simulink model "torqueBalancingStandup"  (Simulink 9.1)
settings: Solver=FixedStepDiscrete  StartTime=0.0  StopTime="Config.SIMULATION_TIME "  FixedStep=Config.Ts  RelTol=1e-3  EnableMultiTasking=on
InitFcn:
  | cd(fileparts(which(bdroot)));
  | initTorqueBalancingStandup;
StopFcn:
  | cd(fileparts(which(bdroot)));
  | stopTorqueBalancingStandup;
undefined symbols (not defined in the file or in its folder): bVectorConstraintsFeet, bVectorConstraintsLegs, Config, ConstraintsMatrixFeet, ConstraintsMatrixLegs, Gain, Reg, ROBOT_DOF, ROBOT_DOF_FOR_SIMULINK, Sat, Sm
libraries: WBToolboxLibrary x95, simulink x4
(part 2 of 2)

== system torqueBalancingStandup/Robot State and References/Select State and References/Visualize Gain Tuning   ==
  smoothingTimeComAndJoints : Inport
  LEFT_RIGHT_FOOT_IN_CONTACT : Inport  Port=2
  impedances : Inport  Port=3
  state : Inport  Port=4
  nu : Inport  Port=5
  Enable : EnablePort
  Demux : Demux  Outputs=2
  Demux1 : Demux  Outputs=Config.numOfJointsForEachControlboard
  Demux2 : Demux  Outputs=Config.numOfJointsForEachControlboard
  Gain : Gain  Gain=180/pi
  Gain1 : Gain  Gain=180/pi
  Impedances(t) : Scope  NumInputPorts=6
  Left right foot in contact : Scope
  Selector1 : Selector  InputPortWidth=6+ROBOT_DOF  IndexOptions=Index vector (dialog)  Indices=[7:6+ROBOT_DOF]  OutputSizes=1
  Selector2 : Selector  InputPortWidth=6+ROBOT_DOF  IndexOptions=Index vector (dialog)  Indices=[1:6]  OutputSizes=1
  jointsSmoothingTime : Scope  NumInputPorts=2
  linear and angular  base velocity : Scope  NumInputPorts=3
  "qjDot(t) " : Scope  NumInputPorts=6
  wires:
  state/1 -> "qjDot(t) "/6, linear and angular  base velocity/3, Impedances(t)/6, jointsSmoothingTime/2  "state"
  LEFT_RIGHT_FOOT_IN_CONTACT/1 -> Left right foot in contact/1  "Left right foot in contact"
  impedances/1 -> Demux1/1
  smoothingTimeComAndJoints/1 -> jointsSmoothingTime/1  "smoothingTimeComAndJoints"
  Demux1/4 -> Impedances(t)/4  "left_leg"
  Demux1/5 -> Impedances(t)/5  "right_leg"
  Demux1/3 -> Impedances(t)/3  "right_arm"
  Demux1/1 -> Impedances(t)/1  "torso"
  Demux1/2 -> Impedances(t)/2  "left_arm"
  Selector1/1 -> Gain/1
  Demux2/4 -> "qjDot(t) "/4  "left_leg"
  Demux2/3 -> "qjDot(t) "/3  "right_arm"
  Demux2/1 -> "qjDot(t) "/1  "torso"
  Demux2/2 -> "qjDot(t) "/2  "left_arm"
  nu/1 -> Selector2/1, Selector1/1
  Selector2/1 -> Demux/1
  Demux/1 -> linear and angular  base velocity/1  "vb"
  Demux/2 -> Gain1/1  "wb"
  Gain/1 -> Demux2/1
  Gain1/1 -> linear and angular  base velocity/2
  Demux2/5 -> "qjDot(t) "/5  "right_leg"

== system torqueBalancingStandup/Robot State and References/State Machine Standup/Compute State Velocity ==
  qj : Inport
  w_H_b : Inport  Port=2
  "feetInContact " : Inport  Port=3
  "state " : Inport  Port=4
  Compute Base Velocity : MATLAB Function  TreatAsAtomicUnit=on
  Fixed Links Jacobians : Subsystem
  Get Measurement : WBToolboxLibrary/wholeBodyStates/Get Measurement  measuredType=Joints Velocity
      settings: SourceProductName=Whole Body Toolbox
  Mux : Mux  Inputs=2
  nu : Outport
  wires:
  Get Measurement/1 -> Mux/2, Compute Base Velocity/4(qjDot)
  Mux/1 -> nu/1
  "feetInContact "/1 -> Compute Base Velocity/3(feetInContact)
  Compute Base Velocity/1(nu_b) -> Mux/1
  Fixed Links Jacobians/1(J_LeftFixed) -> Compute Base Velocity/1(J_LeftFixedLink)
  Fixed Links Jacobians/2(J_RightFixed) -> Compute Base Velocity/2(J_RightFixedLink)
  "state "/1 -> Fixed Links Jacobians/1("state ")
  qj/1 -> Fixed Links Jacobians/2(qj)
  w_H_b/1 -> Fixed Links Jacobians/3(w_H_b)

== system torqueBalancingStandup/Robot State and References/State Machine Standup/Compute base to fixed link transform ==
  qj : Inport
  inertial : Inport  Port=2
  Constant7 : Constant  Value=eye(4)
  "LFoot to base link transform " : Subsystem
  LFoot to world transform (fixed base) : WBToolboxLibrary/wholeBodyModel/Kinematics/Forward Kinematics  frameName=Frames.LEFT_FOOT
      settings: SourceProductName=Whole Body Toolbox
  LLeg to base link transform : Subsystem
  LLeg to world transform (fixed base) : WBToolboxLibrary/wholeBodyModel/Kinematics/Forward Kinematics  frameName=Frames.LEFT_LEG
      settings: SourceProductName=Whole Body Toolbox
  fixed_LFoot_H_b : Outport
  fixed_LLeg_H_b : Outport  Port=2
  wires:
  Constant7/1 -> LLeg to base link transform/4(w_H_base_fixed), "LFoot to base link transform "/4(w_H_base_fixed), LLeg to world transform (fixed base)/1, LFoot to world transform (fixed base)/1
  LLeg to base link transform/1(link_H_b) -> fixed_LLeg_H_b/1
  "LFoot to base link transform "/1(link_H_b) -> fixed_LFoot_H_b/1
  LFoot to world transform (fixed base)/1 -> "LFoot to base link transform "/3(w_H_link)
  LLeg to world transform (fixed base)/1 -> LLeg to base link transform/3(w_H_link)
  qj/1 -> "LFoot to base link transform "/1(qj), LLeg to base link transform/1(qj), LLeg to world transform (fixed base)/2, LFoot to world transform (fixed base)/2
  inertial/1 -> "LFoot to base link transform "/2(inertial), LLeg to base link transform/2(inertial)

== system torqueBalancingStandup/Robot State and References/State Machine Standup/Visualise extrnal wrenches ==
  wL_arm : Inport
  wR_arm : Inport  Port=2
  wL_WBDT : Inport  Port=3
  wR_WBDT : Inport  Port=4
  state : Inport  Port=5
  Enable : EnablePort
  Compute current threshold : MATLAB Function  TreatAsAtomicUnit=on
  Sum : Sum  Inputs=++|
  Sum1 : Sum  Inputs=++|
  left arm ext wrench : Scope  NumInputPorts=3
  left foot ext wrench : Scope  NumInputPorts=3
  right arm ext wrench : Scope  NumInputPorts=3
  right foot ext wrench : Scope  NumInputPorts=3
  sum feet ext wrench : Scope  NumInputPorts=3
  wires:
  wR_WBDT/1 -> Sum/2, right foot ext wrench/1  "wR_WBDT"
  wL_WBDT/1 -> Sum/1, left foot ext wrench/1  "wL_WBDT"
  wR_arm/1 -> right arm ext wrench/1
  wL_arm/1 -> left arm ext wrench/1
  state/1 -> Compute current threshold/1(state), sum feet ext wrench/3, right foot ext wrench/3, left foot ext wrench/3, right arm ext wrench/3, left arm ext wrench/3
  Sum/1 -> sum feet ext wrench/1
  Sum1/1 -> sum feet ext wrench/2
  Compute current threshold/3(thresholdContactLeftFoot) -> left foot ext wrench/2, Sum1/1
  Compute current threshold/4(thresholdContactRightFoot) -> right foot ext wrench/2, Sum1/2
  Compute current threshold/1(thresholdContactLeftHand) -> left arm ext wrench/2
  Compute current threshold/2(thresholdContactRightHand) -> right arm ext wrench/2

== system torqueBalancingStandup/Robot State and References/State Machine Standup/xCom ==
  w_H_b : Inport
  qj : Inport  Port=2
  CoM : WBToolboxLibrary/wholeBodyModel/Kinematics/Forward Kinematics  frameName=Frames.COM
      settings: SourceProductName=Whole Body Toolbox
  "CoM6D ->  CoMXYZ2" : Selector  NumberOfDimensions=2  InputPortWidth=7  IndexOptions=Index vector (dialog),Index vector (dialog)  Indices=[1 2 3],[4]  OutputSizes=1,1
  xCoM : Outport
  wires:
  qj/1 -> CoM/2
  "CoM6D ->  CoMXYZ2"/1 -> xCoM/1
  CoM/1 -> "CoM6D ->  CoMXYZ2"/1
  w_H_b/1 -> CoM/1

== system torqueBalancingStandup/controller_QP/Compute angular momentum integral/Compute base to fixed link transform ==
  qj : Inport
  inertial : Inport  Port=2
  Constant7 : Constant  Value=eye(4)
  "LFoot to base link transform " : Subsystem
  LFoot to world transform (fixed base) : WBToolboxLibrary/wholeBodyModel/Kinematics/Forward Kinematics  frameName=Frames.LEFT_FOOT
      settings: SourceProductName=Whole Body Toolbox
  LLeg to base link transform : Subsystem
  LLeg to world transform (fixed base) : WBToolboxLibrary/wholeBodyModel/Kinematics/Forward Kinematics  frameName=Frames.LEFT_LEG
      settings: SourceProductName=Whole Body Toolbox
  fixed_LLeg_H_b : Outport
  fixed_LFoot_H_b : Outport  Port=2
  wires:
  Constant7/1 -> LLeg to base link transform/4(w_H_base_fixed), "LFoot to base link transform "/4(w_H_base_fixed), LLeg to world transform (fixed base)/1, LFoot to world transform (fixed base)/1
  LLeg to base link transform/1(link_H_b) -> fixed_LLeg_H_b/1
  "LFoot to base link transform "/1(link_H_b) -> fixed_LFoot_H_b/1
  LFoot to world transform (fixed base)/1 -> "LFoot to base link transform "/3(w_H_link)
  LLeg to world transform (fixed base)/1 -> LLeg to base link transform/3(w_H_link)
  qj/1 -> "LFoot to base link transform "/1(qj), LLeg to base link transform/1(qj), LLeg to world transform (fixed base)/2, LFoot to world transform (fixed base)/2
  inertial/1 -> "LFoot to base link transform "/2(inertial), LLeg to base link transform/2(inertial)

== system torqueBalancingStandup/controller_QP/Compute angular momentum integral/Fixed Links Jacobians ==
  "legsInContact " : Inport
  qj : Inport  Port=2
  w_H_b : Inport  Port=3
  " " : WBToolboxLibrary/wholeBodyModel/Jacobians/Jacobian  frameName=Frames.LEFT_LEG
      settings: SourceProductName=Whole Body Toolbox
  "  " : WBToolboxLibrary/wholeBodyModel/Jacobians/Jacobian  frameName=Frames.RIGHT_LEG
      settings: SourceProductName=Whole Body Toolbox
  "   " : WBToolboxLibrary/wholeBodyModel/Jacobians/Jacobian  frameName=Frames.RIGHT_FOOT
      settings: SourceProductName=Whole Body Toolbox
  "       " : WBToolboxLibrary/wholeBodyModel/Jacobians/Jacobian  frameName=Frames.LEFT_FOOT
      settings: SourceProductName=Whole Body Toolbox
  Switch1 : Switch  Criteria=u2 > Threshold  Threshold=0.1
  Switch2 : Switch  Criteria=u2 > Threshold  Threshold=0.1
  J_LeftFixed : Outport
  J_RIghtFixed : Outport  Port=2
  wires:
  Switch2/1 -> J_RIghtFixed/1
  " "/1 -> Switch1/1
  "       "/1 -> Switch1/3
  "   "/1 -> Switch2/3
  "  "/1 -> Switch2/1
  Switch1/1 -> J_LeftFixed/1
  qj/1 -> "   "/2, "  "/2, "       "/2, " "/2
  w_H_b/1 -> "   "/1, " "/1, "       "/1, "  "/1
  "legsInContact "/1 -> Switch2/2, Switch1/2

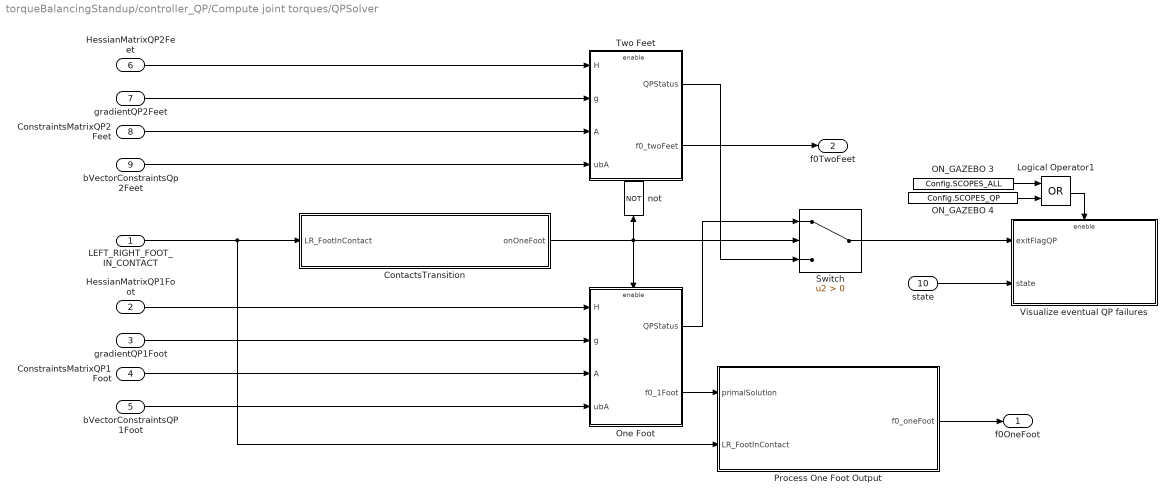
== system torqueBalancingStandup/controller_QP/Compute joint torques/QPSolver ==
  LEFT_RIGHT_FOOT_IN_CONTACT : Inport
  HessianMatrixQP1Foot : Inport  Port=2
  gradientQP1Foot : Inport  Port=3
  ConstraintsMatrixQP1Foot : Inport  Port=4
  bVectorConstraintsQP1Foot : Inport  Port=5
  HessianMatrixQP2Feet : Inport  Port=6
  gradientQP2Feet : Inport  Port=7
  ConstraintsMatrixQP2Feet : Inport  Port=8
  bVectorConstraintsQp2Feet : Inport  Port=9
  state : Inport  Port=10
  ContactsTransition : MATLAB Function  TreatAsAtomicUnit=on
  Logical Operator1 : Logic  Operator=OR  AllPortsSameDT=off  OutDataTypeStr=boolean
  ON_GAZEBO 3 : Constant  Value=Config.SCOPES_ALL
  ON_GAZEBO 4 : Constant  Value=Config.SCOPES_QP
  One Foot : Subsystem  TreatAsAtomicUnit=on
  Process One Foot Output : MATLAB Function  TreatAsAtomicUnit=on
  Switch : Switch  Criteria=u2 > Threshold
  Two Feet : Subsystem  TreatAsAtomicUnit=on
  Visualize eventual QP failures : Subsystem
  not : Logic  Operator=NOT  IconShape=distinctive  AllPortsSameDT=off  OutDataTypeStr=boolean
  f0OneFoot : Outport
  f0TwoFeet : Outport  Port=2
  wires:
  Logical Operator1/1 -> Visualize eventual QP failures/Enable
  state/1 -> Visualize eventual QP failures/2(state)
  LEFT_RIGHT_FOOT_IN_CONTACT/1 -> Process One Foot Output/2(LR_FootInContact), ContactsTransition/1(LR_FootInContact)
  ON_GAZEBO 3/1 -> Logical Operator1/1
  ON_GAZEBO 4/1 -> Logical Operator1/2
  HessianMatrixQP1Foot/1 -> One Foot/1(H)
  bVectorConstraintsQp2Feet/1 -> Two Feet/4(ubA)
  gradientQP1Foot/1 -> One Foot/2(g)
  ConstraintsMatrixQP1Foot/1 -> One Foot/3(A)
  gradientQP2Feet/1 -> Two Feet/2(g)
  ConstraintsMatrixQP2Feet/1 -> Two Feet/3(A)
  not/1 -> Two Feet/Enable
  ContactsTransition/1(onOneFoot) -> One Foot/Enable, Switch/2, not/1
  bVectorConstraintsQP1Foot/1 -> One Foot/4(ubA)
  HessianMatrixQP2Feet/1 -> Two Feet/1(H)
  One Foot/2(f0_1Foot) -> Process One Foot Output/1(primalSolution)
  Process One Foot Output/1(f0_oneFoot) -> f0OneFoot/1
  One Foot/1(QPStatus) -> Switch/1
  Two Feet/1(QPStatus) -> Switch/3
  Switch/1 -> Visualize eventual QP failures/1(exitFlagQP)
  Two Feet/2(f0_twoFeet) -> f0TwoFeet/1

== system torqueBalancingStandup/controller_QP/Compute joint torques (motor reflected inertia)/Check the contribution of feedforward ==
  feedForward : Inport
  u : Inport  Port=2
  Enable : EnablePort
  Demux1 : Demux  Outputs=Config.numOfJointsForEachControlboard
  Demux10 : Demux  Outputs=Config.numOfJointsForEachControlboard
  Demux2 : Demux  Outputs=Config.numOfJointsForEachControlboard
  Sum : Sum  Inputs=|+-
  feedforward_only : Scope  NumInputPorts=5
  u_only : Scope  NumInputPorts=5
  u_with_feedforward : Scope  NumInputPorts=5
  wires:
  Demux10/5 -> u_with_feedforward/5  "right_leg"
  Demux10/2 -> u_with_feedforward/2  "left_arm"
  Demux10/3 -> u_with_feedforward/3  "right_arm"
  Demux10/1 -> u_with_feedforward/1  "torso"
  Demux10/4 -> u_with_feedforward/4  "left_leg"
  Sum/1 -> Demux10/1  "u_with_feedForward"
  feedForward/1 -> Demux1/1, Sum/2
  Demux1/4 -> feedforward_only/4  "left_leg"
  Demux1/5 -> feedforward_only/5  "right_leg"
  Demux1/2 -> feedforward_only/2  "left_arm"
  Demux1/1 -> feedforward_only/1  "torso"
  Demux1/3 -> feedforward_only/3  "right_arm"
  Demux2/4 -> u_only/4  "left_leg"
  Demux2/3 -> u_only/3  "right_arm"
  Demux2/5 -> u_only/5  "right_leg"
  Demux2/2 -> u_only/2  "left_arm"
  u/1 -> Demux2/1, Sum/1
  Demux2/1 -> u_only/1  "torso"

== system torqueBalancingStandup/Robot State and References/Internal Coordinator/Base to fixed_link/LFoot to base link transform  ==
  qj : Inport
  inertial : Inport  Port=2
  w_H_link : Inport  Port=3
  w_H_base_fixed : Inport  Port=4
  Fixed base to imu transform : WBToolboxLibrary/wholeBodyModel/Kinematics/Forward Kinematics  frameName=Frames.IMU
      settings: SourceProductName=Whole Body Toolbox
  Fixed base to root link transform : WBToolboxLibrary/wholeBodyModel/Kinematics/Forward Kinematics  frameName=Frames.BASE
      settings: SourceProductName=Whole Body Toolbox
  Inv\* : Product  Inputs=/*  Multiplication=Matrix(*)
  "Inv\\*  " : Product  Inputs=/*  Multiplication=Matrix(*)
  Neck Position : WBToolboxLibrary/Utilities/Yarp Read  portName=Ports.NECK_POS  signalSize=6  timeout=0.5  blocking=off  timestamp=off  autoconnect=on  errorOnConnection=off
      settings: SourceProductName=Whole Body Toolbox
  Switch6 : Switch  Criteria=u2 > Threshold
  USE_IMU4EST_BASE : Constant  Value=Config.USE_IMU4EST_BASE
  fromImuToHomogeousTransformFCN : MATLAB Function  TreatAsAtomicUnit=on
  holder 1 : WBToolboxLibrary/Utilities/holder 
      settings: SourceProductName=Whole Body Toolbox
  holder 2 : WBToolboxLibrary/Utilities/holder 
      settings: SourceProductName=Whole Body Toolbox
  neck transform : Subsystem
  link_H_b : Outport
  wires:
  Switch6/1 -> link_H_b/1
  "Inv\\*  "/1 -> Switch6/3, fromImuToHomogeousTransformFCN/3(link_H_base)  "link_H_root"
  USE_IMU4EST_BASE/1 -> Switch6/2
  Inv\*/1 -> fromImuToHomogeousTransformFCN/1(imu_H_link), holder 1/1  "imu_H_link"
  holder 2/1 -> fromImuToHomogeousTransformFCN/4(inertial_0)
  Fixed base to imu transform/1 -> Inv\*/1
  holder 1/1 -> fromImuToHomogeousTransformFCN/2(imu_H_link_0)
  qj/1 -> Fixed base to imu transform/2, Fixed base to root link transform/2
  fromImuToHomogeousTransformFCN/1(w_H_b) -> Switch6/1
  Fixed base to root link transform/1 -> "Inv\\*  "/2
  inertial/1 -> holder 2/1, fromImuToHomogeousTransformFCN/5(inertial)
  Neck Position/1 -> neck transform/1(neck port)
  neck transform/1(neck position) -> fromImuToHomogeousTransformFCN/6(neck_pos)
  w_H_link/1 -> "Inv\\*  "/1, Inv\*/2
  w_H_base_fixed/1 -> Fixed base to root link transform/1, Fixed base to imu transform/1

== system torqueBalancingStandup/Robot State and References/Internal Coordinator/Compute State Velocity/Feet Jacobians ==
  qj : Inport
  w_H_b : Inport  Port=2
  Jacobian LFoot : WBToolboxLibrary/wholeBodyModel/Jacobians/Jacobian  frameName=Frames.LEFT_FOOT
      settings: SourceProductName=Whole Body Toolbox
  Jacobian RFoot : WBToolboxLibrary/wholeBodyModel/Jacobians/Jacobian  frameName=Frames.RIGHT_FOOT
      settings: SourceProductName=Whole Body Toolbox
  J_LFoot : Outport
  J_RFoot : Outport  Port=2
  wires:
  Jacobian LFoot/1 -> J_LFoot/1
  Jacobian RFoot/1 -> J_RFoot/1
  w_H_b/1 -> Jacobian RFoot/1, Jacobian LFoot/1
  qj/1 -> Jacobian LFoot/2, Jacobian RFoot/2

== system torqueBalancingStandup/Robot State and References/State Machine Standup/Compute State Velocity/Fixed Links Jacobians ==
  "state " : Inport
  qj : Inport  Port=2
  w_H_b : Inport  Port=3
  " " : WBToolboxLibrary/wholeBodyModel/Jacobians/Jacobian  frameName=Frames.LEFT_LEG
      settings: SourceProductName=Whole Body Toolbox
  "  " : WBToolboxLibrary/wholeBodyModel/Jacobians/Jacobian  frameName=Frames.RIGHT_LEG
      settings: SourceProductName=Whole Body Toolbox
  "   " : WBToolboxLibrary/wholeBodyModel/Jacobians/Jacobian  frameName=Frames.RIGHT_FOOT
      settings: SourceProductName=Whole Body Toolbox
  "       " : WBToolboxLibrary/wholeBodyModel/Jacobians/Jacobian  frameName=Frames.LEFT_FOOT
      settings: SourceProductName=Whole Body Toolbox
  Constant : Constant  Value=Config.iCubStandUp
  Legs in Contact : MATLAB Function  TreatAsAtomicUnit=on
  Switch1 : Switch  Criteria=u2 > Threshold  Threshold=0.1
  Switch2 : Switch  Criteria=u2 > Threshold  Threshold=0.1
  J_LeftFixed : Outport
  J_RightFixed : Outport  Port=2
  wires:
  Switch2/1 -> J_RightFixed/1
  Legs in Contact/1(legsInContact) -> Switch2/2, Switch1/2
  " "/1 -> Switch1/1
  "       "/1 -> Switch1/3
  "   "/1 -> Switch2/3
  "  "/1 -> Switch2/1
  "state "/1 -> Legs in Contact/2(state)
  Constant/1 -> Legs in Contact/1(icubStandup)
  Switch1/1 -> J_LeftFixed/1
  qj/1 -> "   "/2, "  "/2, "       "/2, " "/2
  w_H_b/1 -> "   "/1, " "/1, "       "/1, "  "/1

== system torqueBalancingStandup/Robot State and References/State Machine Standup/Compute base to fixed link transform/LFoot to base link transform  ==
  qj : Inport
  inertial : Inport  Port=2
  w_H_link : Inport  Port=3
  w_H_base_fixed : Inport  Port=4
  Fixed base to imu transform : WBToolboxLibrary/wholeBodyModel/Kinematics/Forward Kinematics  frameName=Frames.IMU
      settings: SourceProductName=Whole Body Toolbox
  Fixed base to root link transform : WBToolboxLibrary/wholeBodyModel/Kinematics/Forward Kinematics  frameName=Frames.BASE
      settings: SourceProductName=Whole Body Toolbox
  Inv\* : Product  Inputs=/*  Multiplication=Matrix(*)
  "Inv\\*  " : Product  Inputs=/*  Multiplication=Matrix(*)
  Neck Position : WBToolboxLibrary/Utilities/Yarp Read  portName=Ports.NECK_POS  signalSize=6  timeout=0.5  blocking=off  timestamp=off  autoconnect=on  errorOnConnection=off
      settings: SourceProductName=Whole Body Toolbox
  Switch6 : Switch  Criteria=u2 > Threshold
  USE_IMU4EST_BASE : Constant  Value=Config.USE_IMU4EST_BASE
  fromImuToHomogeousTransformFCN : MATLAB Function  TreatAsAtomicUnit=on
  holder 1 : WBToolboxLibrary/Utilities/holder 
      settings: SourceProductName=Whole Body Toolbox
  holder 2 : WBToolboxLibrary/Utilities/holder 
      settings: SourceProductName=Whole Body Toolbox
  neck transform : Subsystem
  link_H_b : Outport
  wires:
  Switch6/1 -> link_H_b/1
  "Inv\\*  "/1 -> Switch6/3, fromImuToHomogeousTransformFCN/3(link_H_base)  "link_H_root"
  USE_IMU4EST_BASE/1 -> Switch6/2
  Inv\*/1 -> fromImuToHomogeousTransformFCN/1(imu_H_link), holder 1/1  "imu_H_link"
  holder 2/1 -> fromImuToHomogeousTransformFCN/4(inertial_0)
  Fixed base to imu transform/1 -> Inv\*/1
  holder 1/1 -> fromImuToHomogeousTransformFCN/2(imu_H_link_0)
  qj/1 -> Fixed base to imu transform/2, Fixed base to root link transform/2
  fromImuToHomogeousTransformFCN/1(w_H_b) -> Switch6/1
  Fixed base to root link transform/1 -> "Inv\\*  "/2
  inertial/1 -> holder 2/1, fromImuToHomogeousTransformFCN/5(inertial)
  Neck Position/1 -> neck transform/1(neck port)
  neck transform/1(neck position) -> fromImuToHomogeousTransformFCN/6(neck_pos)
  w_H_link/1 -> "Inv\\*  "/1, Inv\*/2
  w_H_base_fixed/1 -> Fixed base to root link transform/1, Fixed base to imu transform/1

== system torqueBalancingStandup/Robot State and References/State Machine Standup/Compute base to fixed link transform/LLeg to base link transform ==
  qj : Inport
  inertial : Inport  Port=2
  w_H_link : Inport  Port=3
  w_H_base_fixed : Inport  Port=4
  Fixed base to imu transform : WBToolboxLibrary/wholeBodyModel/Kinematics/Forward Kinematics  frameName=Frames.IMU
      settings: SourceProductName=Whole Body Toolbox
  Fixed base to root link transform : WBToolboxLibrary/wholeBodyModel/Kinematics/Forward Kinematics  frameName=Frames.BASE
      settings: SourceProductName=Whole Body Toolbox
  Inv\* : Product  Inputs=/*  Multiplication=Matrix(*)
  "Inv\\*  " : Product  Inputs=/*  Multiplication=Matrix(*)
  Neck Position : WBToolboxLibrary/Utilities/Yarp Read  portName=Ports.NECK_POS  signalSize=6  timeout=0.5  blocking=off  timestamp=off  autoconnect=on  errorOnConnection=off
      settings: SourceProductName=Whole Body Toolbox
  Switch6 : Switch  Criteria=u2 > Threshold
  USE_IMU4EST_BASE : Constant  Value=Config.USE_IMU4EST_BASE
  fromImuToHomogeousTransformFCN : MATLAB Function  TreatAsAtomicUnit=on
  holder 1 : WBToolboxLibrary/Utilities/holder 
      settings: SourceProductName=Whole Body Toolbox
  holder 2 : WBToolboxLibrary/Utilities/holder 
      settings: SourceProductName=Whole Body Toolbox
  neck transform : Subsystem
  link_H_b : Outport
  wires:
  Switch6/1 -> link_H_b/1
  "Inv\\*  "/1 -> Switch6/3, fromImuToHomogeousTransformFCN/3(link_H_base)  "link_H_root"
  USE_IMU4EST_BASE/1 -> Switch6/2
  Inv\*/1 -> fromImuToHomogeousTransformFCN/1(imu_H_link), holder 1/1  "imu_H_link"
  holder 2/1 -> fromImuToHomogeousTransformFCN/4(inertial_0)
  Fixed base to imu transform/1 -> Inv\*/1
  holder 1/1 -> fromImuToHomogeousTransformFCN/2(imu_H_link_0)
  qj/1 -> Fixed base to imu transform/2, Fixed base to root link transform/2
  fromImuToHomogeousTransformFCN/1(w_H_b) -> Switch6/1
  Fixed base to root link transform/1 -> "Inv\\*  "/2
  inertial/1 -> holder 2/1, fromImuToHomogeousTransformFCN/5(inertial)
  Neck Position/1 -> neck transform/1(neck port)
  neck transform/1(neck position) -> fromImuToHomogeousTransformFCN/6(neck_pos)
  w_H_link/1 -> "Inv\\*  "/1, Inv\*/2
  w_H_base_fixed/1 -> Fixed base to root link transform/1, Fixed base to imu transform/1

== system torqueBalancingStandup/controller_QP/Compute angular momentum integral/Compute base to fixed link transform/LFoot to base link transform  ==
  qj : Inport
  inertial : Inport  Port=2
  w_H_link : Inport  Port=3
  w_H_base_fixed : Inport  Port=4
  Fixed base to imu transform : WBToolboxLibrary/wholeBodyModel/Kinematics/Forward Kinematics  frameName=Frames.IMU
      settings: SourceProductName=Whole Body Toolbox
  Fixed base to root link transform : WBToolboxLibrary/wholeBodyModel/Kinematics/Forward Kinematics  frameName=Frames.BASE
      settings: SourceProductName=Whole Body Toolbox
  Inv\* : Product  Inputs=/*  Multiplication=Matrix(*)
  "Inv\\*  " : Product  Inputs=/*  Multiplication=Matrix(*)
  Neck Position : WBToolboxLibrary/Utilities/Yarp Read  portName=Ports.NECK_POS  signalSize=6  timeout=0.5  blocking=off  timestamp=off  autoconnect=on  errorOnConnection=off
      settings: SourceProductName=Whole Body Toolbox
  Switch6 : Switch  Criteria=u2 > Threshold
  USE_IMU4EST_BASE : Constant  Value=Config.USE_IMU4EST_BASE
  fromImuToHomogeousTransformFCN : MATLAB Function  TreatAsAtomicUnit=on
  holder 1 : WBToolboxLibrary/Utilities/holder 
      settings: SourceProductName=Whole Body Toolbox
  holder 2 : WBToolboxLibrary/Utilities/holder 
      settings: SourceProductName=Whole Body Toolbox
  neck transform : Subsystem
  link_H_b : Outport
  wires:
  Switch6/1 -> link_H_b/1
  "Inv\\*  "/1 -> Switch6/3, fromImuToHomogeousTransformFCN/3(link_H_base)  "link_H_root"
  USE_IMU4EST_BASE/1 -> Switch6/2
  Inv\*/1 -> fromImuToHomogeousTransformFCN/1(imu_H_link), holder 1/1  "imu_H_link"
  holder 2/1 -> fromImuToHomogeousTransformFCN/4(inertial_0)
  Fixed base to imu transform/1 -> Inv\*/1
  holder 1/1 -> fromImuToHomogeousTransformFCN/2(imu_H_link_0)
  qj/1 -> Fixed base to imu transform/2, Fixed base to root link transform/2
  fromImuToHomogeousTransformFCN/1(w_H_b) -> Switch6/1
  Fixed base to root link transform/1 -> "Inv\\*  "/2
  inertial/1 -> holder 2/1, fromImuToHomogeousTransformFCN/5(inertial)
  Neck Position/1 -> neck transform/1(neck port)
  neck transform/1(neck position) -> fromImuToHomogeousTransformFCN/6(neck_pos)
  w_H_link/1 -> "Inv\\*  "/1, Inv\*/2
  w_H_base_fixed/1 -> Fixed base to root link transform/1, Fixed base to imu transform/1

== system torqueBalancingStandup/controller_QP/Compute angular momentum integral/Compute base to fixed link transform/LLeg to base link transform ==
  qj : Inport
  inertial : Inport  Port=2
  w_H_link : Inport  Port=3
  w_H_base_fixed : Inport  Port=4
  Fixed base to imu transform : WBToolboxLibrary/wholeBodyModel/Kinematics/Forward Kinematics  frameName=Frames.IMU
      settings: SourceProductName=Whole Body Toolbox
  Fixed base to root link transform : WBToolboxLibrary/wholeBodyModel/Kinematics/Forward Kinematics  frameName=Frames.BASE
      settings: SourceProductName=Whole Body Toolbox
  Inv\* : Product  Inputs=/*  Multiplication=Matrix(*)
  "Inv\\*  " : Product  Inputs=/*  Multiplication=Matrix(*)
  Neck Position : WBToolboxLibrary/Utilities/Yarp Read  portName=Ports.NECK_POS  signalSize=6  timeout=0.5  blocking=off  timestamp=off  autoconnect=on  errorOnConnection=off
      settings: SourceProductName=Whole Body Toolbox
  Switch6 : Switch  Criteria=u2 > Threshold
  USE_IMU4EST_BASE : Constant  Value=Config.USE_IMU4EST_BASE
  fromImuToHomogeousTransformFCN : MATLAB Function  TreatAsAtomicUnit=on
  holder 1 : WBToolboxLibrary/Utilities/holder 
      settings: SourceProductName=Whole Body Toolbox
  holder 2 : WBToolboxLibrary/Utilities/holder 
      settings: SourceProductName=Whole Body Toolbox
  neck transform : Subsystem
  link_H_b : Outport
  wires:
  Switch6/1 -> link_H_b/1
  "Inv\\*  "/1 -> Switch6/3, fromImuToHomogeousTransformFCN/3(link_H_base)  "link_H_root"
  USE_IMU4EST_BASE/1 -> Switch6/2
  Inv\*/1 -> fromImuToHomogeousTransformFCN/1(imu_H_link), holder 1/1  "imu_H_link"
  holder 2/1 -> fromImuToHomogeousTransformFCN/4(inertial_0)
  Fixed base to imu transform/1 -> Inv\*/1
  holder 1/1 -> fromImuToHomogeousTransformFCN/2(imu_H_link_0)
  qj/1 -> Fixed base to imu transform/2, Fixed base to root link transform/2
  fromImuToHomogeousTransformFCN/1(w_H_b) -> Switch6/1
  Fixed base to root link transform/1 -> "Inv\\*  "/2
  inertial/1 -> holder 2/1, fromImuToHomogeousTransformFCN/5(inertial)
  Neck Position/1 -> neck transform/1(neck port)
  neck transform/1(neck position) -> fromImuToHomogeousTransformFCN/6(neck_pos)
  w_H_link/1 -> "Inv\\*  "/1, Inv\*/2
  w_H_base_fixed/1 -> Fixed base to root link transform/1, Fixed base to imu transform/1

== system torqueBalancingStandup/controller_QP/Compute joint torques/QPSolver/One Foot ==
  H : Inport
  g : Inport  Port=2
  A : Inport  Port=3
  ubA : Inport  Port=4
  Enable : EnablePort
  Analytical Solution One Foot (unconstrained) : MATLAB Function  TreatAsAtomicUnit=on
  Match Signal Sizes1 : WBToolboxLibrary/Utilities/Match Signal Sizes
      settings: SourceProductName=Whole Body Toolbox
  Process QP output : MATLAB Function  TreatAsAtomicUnit=on
  QP Two Feet : WBToolboxLibrary/Utilities/QP  lbA=off  ubA=on  lb=off  ub=off  computeObjVal=off  stopIfFails=off
      settings: SourceProductName=Whole Body Toolbox
  QPStatus : Outport
  f0_1Foot : Outport  Port=2
  wires:
  H/1 -> Analytical Solution One Foot (unconstrained)/1(H), QP Two Feet/1
  ubA/1 -> QP Two Feet/4
  A/1 -> QP Two Feet/3
  QP Two Feet/2 -> Process QP output/3(QPStatus), QPStatus/1
  QP Two Feet/1 -> Match Signal Sizes1/2
  g/1 -> Analytical Solution One Foot (unconstrained)/2(g), Match Signal Sizes1/1, QP Two Feet/2
  Match Signal Sizes1/1 -> Process QP output/2(primalSolution)
  Analytical Solution One Foot (unconstrained)/1(analyticalSolution) -> Process QP output/1(analyticalSolution)
  Process QP output/1(f0) -> f0_1Foot/1

== system torqueBalancingStandup/controller_QP/Compute joint torques/QPSolver/Two Feet ==
  H : Inport
  g : Inport  Port=2
  A : Inport  Port=3
  ubA : Inport  Port=4
  Enable : EnablePort
  Analytical Solution Two Feet (unconstrained) : MATLAB Function  TreatAsAtomicUnit=on
  Match Signal Sizes : WBToolboxLibrary/Utilities/Match Signal Sizes
      settings: SourceProductName=Whole Body Toolbox
  Process QP output : MATLAB Function  TreatAsAtomicUnit=on
  QP Two Feet : WBToolboxLibrary/Utilities/QP  lbA=off  ubA=on  lb=off  ub=off  computeObjVal=off  stopIfFails=off
      settings: SourceProductName=Whole Body Toolbox
  QPStatus : Outport
  f0_twoFeet : Outport  Port=2
  wires:
  H/1 -> QP Two Feet/1, Analytical Solution Two Feet (unconstrained)/1(H)
  ubA/1 -> QP Two Feet/4
  A/1 -> QP Two Feet/3
  g/1 -> Analytical Solution Two Feet (unconstrained)/2(g), Match Signal Sizes/1, QP Two Feet/2
  QP Two Feet/2 -> QPStatus/1, Process QP output/3(QPStatus)
  QP Two Feet/1 -> Match Signal Sizes/2
  Match Signal Sizes/1 -> Process QP output/2(primalSolution)
  Analytical Solution Two Feet (unconstrained)/1(analyticalSolution) -> Process QP output/1(analyticalSolution)
  Process QP output/1(f0) -> f0_twoFeet/1

== system torqueBalancingStandup/controller_QP/Compute joint torques/QPSolver/Visualize eventual QP failures ==
  exitFlagQP : Inport
  state : Inport  Port=2
  Enable : EnablePort
  "QP status (0: no failure, 1: not using)" : Scope  NumInputPorts=2
  wires:
  exitFlagQP/1 -> "QP status (0: no failure, 1: not using)"/1  "exitFlagQP"
  state/1 -> "QP status (0: no failure, 1: not using)"/2

== system torqueBalancingStandup/Robot State and References/Internal Coordinator/Base to fixed_link/LFoot to base link transform /neck transform ==
  neck port : Inport
  Constant : Constant  Value=zeros(3,1)
  Gain : Gain  Gain=pi/180
  Selector1 : Selector  InputPortWidth=6  IndexOptions=Index vector (dialog)  Indices=[1:3]  OutputSizes=1
  Switch : Switch  Criteria=u2 > Threshold
  USE_IMU4EST_BASE1 : Constant  Value=Config.CORRECT_NECK_IMU
  neck position : Outport
  wires:
  neck port/1 -> Gain/1
  USE_IMU4EST_BASE1/1 -> Switch/2
  Switch/1 -> neck position/1
  Gain/1 -> Selector1/1
  Constant/1 -> Switch/3
  Selector1/1 -> Switch/1  "neck pos"

== system torqueBalancingStandup/Robot State and References/State Machine Standup/Compute base to fixed link transform/LFoot to base link transform /neck transform ==
  neck port : Inport
  Constant : Constant  Value=zeros(3,1)
  Gain : Gain  Gain=pi/180
  Selector1 : Selector  InputPortWidth=6  IndexOptions=Index vector (dialog)  Indices=[1:3]  OutputSizes=1
  Switch : Switch  Criteria=u2 > Threshold
  USE_IMU4EST_BASE1 : Constant  Value=Config.CORRECT_NECK_IMU
  neck position : Outport
  wires:
  neck port/1 -> Gain/1
  USE_IMU4EST_BASE1/1 -> Switch/2
  Switch/1 -> neck position/1
  Gain/1 -> Selector1/1
  Constant/1 -> Switch/3
  Selector1/1 -> Switch/1  "neck pos"

== system torqueBalancingStandup/Robot State and References/State Machine Standup/Compute base to fixed link transform/LLeg to base link transform/neck transform ==
  neck port : Inport
  Constant : Constant  Value=zeros(3,1)
  Gain : Gain  Gain=pi/180
  Selector1 : Selector  InputPortWidth=6  IndexOptions=Index vector (dialog)  Indices=[1:3]  OutputSizes=1
  Switch : Switch  Criteria=u2 > Threshold
  USE_IMU4EST_BASE1 : Constant  Value=Config.CORRECT_NECK_IMU
  neck position : Outport
  wires:
  neck port/1 -> Gain/1
  USE_IMU4EST_BASE1/1 -> Switch/2
  Switch/1 -> neck position/1
  Gain/1 -> Selector1/1
  Constant/1 -> Switch/3
  Selector1/1 -> Switch/1  "neck pos"

== system torqueBalancingStandup/controller_QP/Compute angular momentum integral/Compute base to fixed link transform/LFoot to base link transform /neck transform ==
  neck port : Inport
  Constant : Constant  Value=zeros(3,1)
  Gain : Gain  Gain=pi/180
  Selector1 : Selector  InputPortWidth=6  IndexOptions=Index vector (dialog)  Indices=[1:3]  OutputSizes=1
  Switch : Switch  Criteria=u2 > Threshold
  USE_IMU4EST_BASE1 : Constant  Value=Config.CORRECT_NECK_IMU
  neck position : Outport
  wires:
  neck port/1 -> Gain/1
  USE_IMU4EST_BASE1/1 -> Switch/2
  Switch/1 -> neck position/1
  Gain/1 -> Selector1/1
  Constant/1 -> Switch/3
  Selector1/1 -> Switch/1  "neck pos"

== system torqueBalancingStandup/controller_QP/Compute angular momentum integral/Compute base to fixed link transform/LLeg to base link transform/neck transform ==
  neck port : Inport
  Constant : Constant  Value=zeros(3,1)
  Gain : Gain  Gain=pi/180
  Selector1 : Selector  InputPortWidth=6  IndexOptions=Index vector (dialog)  Indices=[1:3]  OutputSizes=1
  Switch : Switch  Criteria=u2 > Threshold
  USE_IMU4EST_BASE1 : Constant  Value=Config.CORRECT_NECK_IMU
  neck position : Outport
  wires:
  neck port/1 -> Gain/1
  USE_IMU4EST_BASE1/1 -> Switch/2
  Switch/1 -> neck position/1
  Gain/1 -> Selector1/1
  Constant/1 -> Switch/3
  Selector1/1 -> Switch/1  "neck pos"

== matlab function controller_QP/Compute angular momentum integral/Compute base to fixed link transform/LFoot to base link transform /fromImuToHomogeousTransformFCN ==
  data: imu_H_link input double; imu_H_link_0 input double; link_H_base input double; inertial_0 input double; inertial input double; neck_pos input double; w_H_b output double; Config parameter double
function w_H_b = worldToBaseTransformWithIMUFCN(imu_H_link,imu_H_link_0,link_H_base,inertial_0,inertial,neck_pos,Config)

    w_H_b = worldToBaseTransformWithIMU(imu_H_link,imu_H_link_0,link_H_base,inertial_0,inertial,neck_pos,Config);

end

== matlab function Robot State and References/Internal Coordinator/Base to fixed_link/LFoot to base link transform /fromImuToHomogeousTransformFCN ==
  data: imu_H_link input double; imu_H_link_0 input double; link_H_base input double; inertial_0 input double; inertial input double; neck_pos input double; w_H_b output double; Config parameter double
function w_H_b = worldToBaseTransformWithIMUFCN(imu_H_link,imu_H_link_0,link_H_base,inertial_0,inertial,neck_pos,Config)

    w_H_b = worldToBaseTransformWithIMU(imu_H_link,imu_H_link_0,link_H_base,inertial_0,inertial,neck_pos,Config);

end

== matlab function Robot State and References/State Machine Standup/Compute base to fixed link transform/LLeg to base link transform/fromImuToHomogeousTransformFCN ==
  data: imu_H_link input double; imu_H_link_0 input double; link_H_base input double; inertial_0 input double; inertial input double; neck_pos input double; w_H_b output double; Config parameter double
function w_H_b = worldToBaseTransformWithIMUFCN(imu_H_link,imu_H_link_0,link_H_base,inertial_0,inertial,neck_pos,Config)

    w_H_b = worldToBaseTransformWithIMU(imu_H_link,imu_H_link_0,link_H_base,inertial_0,inertial,neck_pos,Config);

end

== matlab function controller_QP/Compute angular momentum integral/Compute base to fixed link transform/LLeg to base link transform/fromImuToHomogeousTransformFCN ==
  data: imu_H_link input double; imu_H_link_0 input double; link_H_base input double; inertial_0 input double; inertial input double; neck_pos input double; w_H_b output double; Config parameter double
function w_H_b = worldToBaseTransformWithIMUFCN(imu_H_link,imu_H_link_0,link_H_base,inertial_0,inertial,neck_pos,Config)

    w_H_b = worldToBaseTransformWithIMU(imu_H_link,imu_H_link_0,link_H_base,inertial_0,inertial,neck_pos,Config);

end

== matlab function Robot State and References/Internal Coordinator/Compute State Velocity/Compute Base Velocity ==
  data: J_LeftFoot input double; J_RightFoot input double; feetInContact input double; nu_b output double; qjDot input double; Reg parameter double
function nu_b = computeBaseVelocityFCN(J_LeftFoot, J_RightFoot, feetInContact, qjDot, Reg)

    nu_b = computeBaseVelocity(J_LeftFoot, J_RightFoot, feetInContact, qjDot, Reg);
end

== matlab function Dynamics and Kinematics/Dynamics/Add motors reflected inertias/Add motor reflected inertias ==
  data: M input double; M_with_inertia output double; Config parameter double
function M_with_inertia = addMotorsInertiaFCN(M,Config)

    M_with_inertia = addMotorsInertia(M,Config);

end

== matlab function Robot State and References/State Machine Standup/Compute State Velocity/Compute Base Velocity ==
  data: J_LeftFixedLink input double; J_RightFixedLink input double; feetInContact input double; nu_b output double; qjDot input double; Reg parameter double
function nu_b = computeBaseVelocityFCN(J_LeftFixedLink, J_RightFixedLink, feetInContact, qjDot, Reg)

    nu_b = computeBaseVelocity(J_LeftFixedLink, J_RightFixedLink, feetInContact, qjDot, Reg);
end

== matlab function Robot State and References/State Machine Standup/Compute base to fixed link transform/LFoot to base link transform /fromImuToHomogeousTransformFCN ==
  data: imu_H_link input double; imu_H_link_0 input double; link_H_base input double; inertial_0 input double; inertial input double; neck_pos input double; w_H_b output double; Config parameter double
function w_H_b = worldToBaseTransformWithIMUFCN(imu_H_link,imu_H_link_0,link_H_base,inertial_0,inertial,neck_pos,Config)

    w_H_b = worldToBaseTransformWithIMU(imu_H_link,imu_H_link_0,link_H_base,inertial_0,inertial,neck_pos,Config);

end

== matlab function Dynamics and Kinematics/Kinematics/Legs in Contact ==
  data: icubStandup input double; legsInContact output double; state input double
function legsInContact = legsContactDetectorFCN(icubStandup,state)

   legsInContact = legsContactDetector(icubStandup,state);
end

== matlab function Robot State and References/Internal Coordinator/Reference Generator CoM ==
  data: pos_CoM_0 input double; t input double; references_CoM output double; Config parameter double
function references_CoM = referenceGeneratorCoMFCN(pos_CoM_0, t, Config)

    references_CoM = referenceGeneratorCoM(pos_CoM_0, t, Config);
end

== matlab function controller_QP/Compute angular momentum integral/Legs in Contact ==
  data: icubStandup input double; legsInContact output double; state input double
function legsInContact = legsContactDetectorFCN(icubStandup,state)

   legsInContact = legsContactDetector(icubStandup,state);
end

== matlab function controller_QP/Compute joint torques (motor reflected inertia)/(transpose(T*Gamma))^{-1}*I_m*(T*Gamma)^{-1} ==
  data: reflectedInertia output double; Config parameter double
function reflectedInertia  = computeMotorsInertiaFCN(Config)

    [reflectedInertia] = computeMotorsInertia(Config);

end

== matlab function Robot State and References/State Machine Standup/stateMachineStandupFCN ==
  data: wrench_rightFoot input double; wrench_leftFoot input double; w_H_b output double; constraints output double; CoM_des output double; qj_des output double; wrench_leftHand input double; wrench_rightHand input double; xCoM_0 input double; qj_0 input double; xCoM input double; l_sole_H_b input double; l_upper_leg_contact_H_b input double; t input double; STANDUP_WITH_HUMAN input double; Sm parameter double; impedances output double; KPCoM output double; KDCoM output double; Gain parameter double; currentState output double; jointsAndCoMSmoothingTime output double
function [w_H_b, constraints, CoM_des, qj_des, impedances, KPCoM, KDCoM, currentState, jointsAndCoMSmoothingTime] = ...
             stateMachineStandupFCN(wrench_rightFoot, wrench_leftFoot, wrench_leftHand, wrench_rightHand, xCoM_0, qj_0, xCoM, l_sole_H_b, l_upper_leg_contact_H_b, t, STANDUP_WITH_HUMAN, Sm, Gain)
         
         [w_H_b, constraints, CoM_des, qj_des, impedances, KPCoM, KDCoM, currentState, jointsAndCoMSmoothingTime] = ...
             stateMachineStandup(wrench_rightFoot, wrench_leftFoot, wrench_leftHand, wrench_rightHand, xCoM_0, qj_0, xCoM, l_sole_H_b, l_upper_leg_contact_H_b, t, STANDUP_WITH_HUMAN, Sm, Gain);
end

== matlab function Robot State and References/State Machine Standup/Compute State Velocity/Fixed Links Jacobians/Legs in Contact ==
  data: icubStandup input double; legsInContact output double; state input double
function legsInContact = legsContactDetectorFCN(icubStandup,state)

   legsInContact = legsContactDetector(icubStandup,state);
end

== matlab function controller_QP/Compute joint torques/QPSolver/ContactsTransition ==
  data: LR_FootInContact input double; onOneFoot output double
function onOneFoot = contactsTransitionQPFCN(LR_FootInContact)

    onOneFoot = contactsTransitionQP(LR_FootInContact);
end

== matlab function controller_QP/Compute joint torques/QPSolver/Process One Foot Output ==
  data: primalSolution input double; f0_oneFoot output double; LR_FootInContact input double
function f0_oneFoot = processOneFootOutputQPFCN(primalSolution,LR_FootInContact)

    f0_oneFoot = processOneFootOutputQP(primalSolution,LR_FootInContact);
end

== matlab function controller_QP/Balancing Controller  ==
  data: tauModel output double; Sigma output double; NA output double; f_LDot output double; HessianMatrixQP1Foot output double; gradientQP1Foot output double; ConstraintsMatrixQP1Foot output double; bVectorConstraintsQp1Foot output double; HessianMatrixQP2FeetOrLegs output double; gradientQP2FeetOrLegs output double; ConstraintsMatrixQP2FeetOrLegs output double; bVectorConstraintsQp2FeetOrLegs output double; constraints input double; ROBOT_DOF_FOR_SIMULINK input double; ConstraintsMatrix input double; bVectorConstraints input double; qj input double; qjDes input double; nu input double; M input double; h input double; L input double; intLw input double; w_H_l_contact input double; w_H_r_contact input double; JL input double; JR input double; dJL_nu input double; dJR_nu input double; xCoM input double; J_CoM input double; desired_x_dx_ddx_CoM input double; gainsPCOM input double; gainsDCOM input double; impedances input double; Reg parameter double; errorCoM output double; f_noQP output double; Gain parameter double; w_H_lArm input double; w_H_rArm input double; LArmWrench input double; RArmWrench input double; STANDUP_WITH_HUMAN input double; correctionFromSupportForce output double; L_error output double; V output double; state input double
function [tauModel, Sigma, NA, f_LDot, ...
          HessianMatrixQP1Foot, gradientQP1Foot, ConstraintsMatrixQP1Foot, bVectorConstraintsQp1Foot, ...
          HessianMatrixQP2FeetOrLegs, gradientQP2FeetOrLegs, ConstraintsMatrixQP2FeetOrLegs, bVectorConstraintsQp2FeetOrLegs, ...
          errorCoM, f_noQP, correctionFromSupportForce, L_error, V] =  ...
              balancingControllerStandupFCN(constraints, ROBOT_DOF_FOR_SIMULINK, ConstraintsMatrix, bVectorConstraints, ...
                                            qj, qjDes, nu, M, h, L, intLw, w_H_l_contact, w_H_r_contact, JL, JR, dJL_nu, dJR_nu, xCoM, J_CoM, desired_x_dx_ddx_CoM, ...
                                            gainsPCOM, gainsDCOM, impedances, Reg, Gain, w_H_lArm, w_H_rArm, LArmWrench, RArmWrench, STANDUP_WITH_HUMAN, state)
           
   [tauModel, Sigma, NA, f_LDot, ...
          HessianMatrixQP1Foot, gradientQP1Foot, ConstraintsMatrixQP1Foot, bVectorConstraintsQp1Foot, ...
          HessianMatrixQP2FeetOrLegs, gradientQP2FeetOrLegs, ConstraintsMatrixQP2FeetOrLegs, bVectorConstraintsQp2FeetOrLegs, ...
          errorCoM, f_noQP, correctionFromSupportForce, L_error, V] =  ...
              balancingControllerStandup(constraints, ROBOT_DOF_FOR_SIMULINK, ConstraintsMatrix, bVectorConstraints, ...
                                         qj, qjDes, nu, M, h, L, intLw, w_H_l_contact, w_H_r_contact, JL, JR, dJL_nu, dJR_nu, xCoM, J_CoM, desired_x_dx_ddx_CoM, ...
                                         gainsPCOM, gainsDCOM, impedances, Reg, Gain, w_H_lArm, w_H_rArm, LArmWrench, RArmWrench, STANDUP_WITH_HUMAN, state);
end

== matlab function emergency stop: joint limits/MATLAB Function ==
  data: umin input double; umax input double; u input double; inRange output double; tol input double
function inRange = checkRangeFCN(umin, umax, u, tol)

    inRange = checkRange(umin, umax, u, tol);
end

== matlab function controller_QP/Compute joint torques/QPSolver/One Foot/Process QP output ==
  data: analyticalSolution input double; primalSolution input double; QPStatus input double; f0 output double; Config parameter double
function f0 = processOutputQPFCN(analyticalSolution,primalSolution,QPStatus,Config)

     f0 = processOutputQP(analyticalSolution,primalSolution,QPStatus,Config);
end

== matlab function controller_QP/Compute angular momentum integral/References for L ==
  data: qjErr input double; JL input double; JR input double; nu_b_equivalent output double; Reg parameter double; activeFeetConstraints input double
function nu_b_equivalent = generateReferencesForH_FCN(qjErr, JL, JR, Reg, activeFeetConstraints)

    if activeFeetConstraints(1) == 1
    
        pinvJb          = (JL(:,1:6)'*JL(:,1:6) + Reg.pinvDamp_nu_b*eye(6))\JL(:,1:6)';
        nu_b_equivalent = -pinvJb*JL(:,7:end)*qjErr;
    else
    
        pinvJb          = (JR(:,1:6)'*JR(:,1:6) + Reg.pinvDamp_nu_b*eye(6))\JR(:,1:6)';
        nu_b_equivalent = -pinvJb*JR(:,7:end)*qjErr;
    end
end

== matlab function controller_QP/Compute joint torques/QPSolver/Two Feet/Analytical Solution Two Feet (unconstrained) ==
  data: H input double; analyticalSolution output double; g input double
function analyticalSolution = analyticalSolutionQPFCN(H,g)

    analyticalSolution = analyticalSolutionQP(H,g);
end

== matlab function controller_QP/Compute joint torques/QPSolver/One Foot/Analytical Solution One Foot (unconstrained) ==
  data: H input double; analyticalSolution output double; g input double
function analyticalSolution = analyticalSolutionQPFCN(H,g)

    analyticalSolution = analyticalSolutionQP(H,g);
end

== matlab function controller_QP/Compute joint torques/QPSolver/Two Feet/Process QP output ==
  data: analyticalSolution input double; primalSolution input double; QPStatus input double; f0 output double; Config parameter double
function f0 = processOutputQPFCN(analyticalSolution,primalSolution,QPStatus,Config)

     f0 = processOutputQP(analyticalSolution,primalSolution,QPStatus,Config);
end

== matlab function Robot State and References/State Machine Standup/Visualise extrnal wrenches/Compute current threshold ==
  data: thresholdContactLeftHand output double; thresholdContactRightHand output double; state input double; thresholdContactLeftFoot output double; thresholdContactRightFoot output double; Sm parameter double
function [thresholdContactLeftHand,thresholdContactRightHand, ...
          thresholdContactLeftFoot,thresholdContactRightFoot] = currentThreshold(state,Sm)

    thresholdContactLeftHand  = Sm.wrench_thresholdContactLHand(state);
    thresholdContactRightHand = Sm.wrench_thresholdContactRHand(state);
    thresholdContactLeftFoot  = Sm.wrench_thresholdContactLFoot(state);
    thresholdContactRightFoot = Sm.wrench_thresholdContactRFoot(state);
end
